simulink model "Halvorsen"  (R2014b)
settings: Solver=ode45  StartTime=0.0  StopTime=10.0  RelTol=1e-3
values from neighbouring files (symbols this model uses):
  a = 0.95    [Run_Aizawa.m]    (also in Run_Arneodo.m = -5.5; Run_Chen.m = 33; Run_Chua.m = 15.6; Run_Chua_4D.m = 0.03)
undefined symbols (not defined in the file or in its folder): param
settings Model: Creator=Arek  LastModifiedBy=Arek

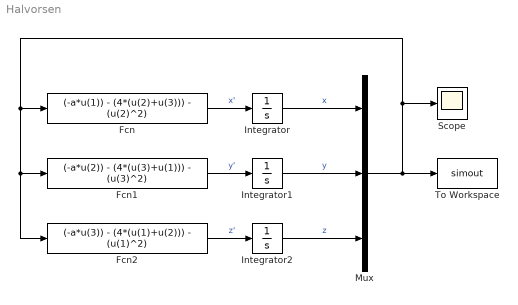
== system Halvorsen ==
  Fcn : Fcn  Expr=(-a*u(1)) - (4*(u(2)+u(3))) - (u(2)^2)
  Fcn1 : Fcn  Expr=(-a*u(2)) - (4*(u(3)+u(1))) - (u(3)^2)
  Fcn2 : Fcn  Expr=(-a*u(3)) - (4*(u(1)+u(2))) - (u(1)^2)
  Integrator : Integrator  InitialCondition=param.ic(1)
  Integrator1 : Integrator  InitialCondition=param.ic(2)
  Integrator2 : Integrator  InitialCondition=param.ic(3)
  Mux : Mux  Inputs=3
  Scope : Scope
      settings: ShowLegends=on
  To Workspace : ToWorkspace  VariableName=simout  SaveFormat=Timeseries  SampleTime=-1
  wires:
  Fcn/1 -> Integrator/1  "x'"
  Integrator/1 -> Mux/1  "x"
  Fcn1/1 -> Integrator1/1  "y'"
  Integrator1/1 -> Mux/2  "y"
  Fcn2/1 -> Integrator2/1  "z'"
  Integrator2/1 -> Mux/3  "z"
  Mux/1 -> Fcn/1, Fcn1/1, Fcn2/1, Scope/1, To Workspace/1
